simulink model "DynamicModelRacingWind"  (R2016b)
settings: configuration reference "WheelSimConfiguration2016" (kept outside this file)
settings Model: Creator=At  LastModifiedBy=At
settings ConfigSetRef: SourceLocation=Base Workspace

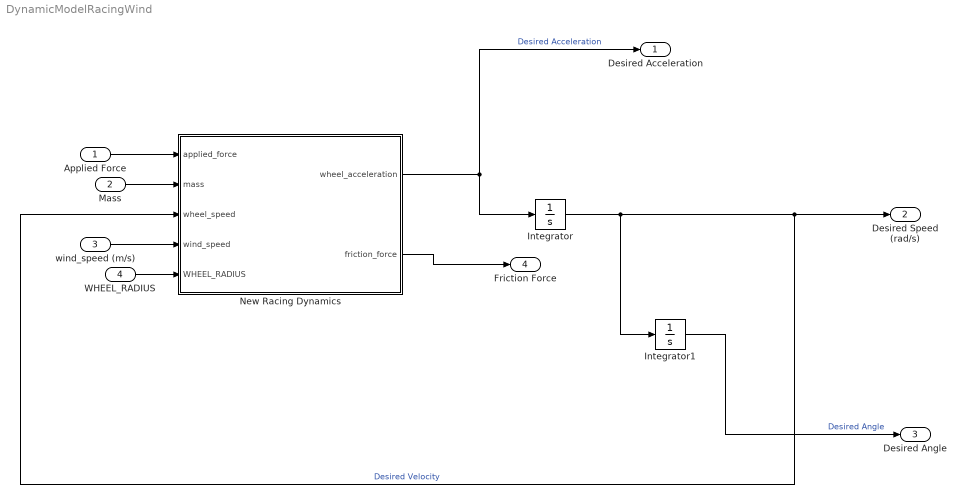
== system DynamicModelRacingWind ==
  Applied Force : Inport
  Mass : Inport  Port=2
  wind_speed (m/s) : Inport  Port=3
  WHEEL_RADIUS : Inport  Port=4
  Integrator : Integrator
  Integrator1 : Integrator
  New Racing Dynamics : MATLAB Function  TreatAsAtomicUnit=on
  Desired Acceleration : Outport
  Desired Speed (rad/s) : Outport  Port=2
  Desired Angle : Outport  Port=3
  Friction Force : Outport  Port=4
  wires:
  New Racing Dynamics/1(wheel_acceleration) -> Integrator/1, Desired Acceleration/1  "Desired Acceleration"
  Integrator/1 -> Desired Speed (rad/s)/1, New Racing Dynamics/3(wheel_speed), Integrator1/1  "Desired Velocity"
  Integrator1/1 -> Desired Angle/1  "Desired Angle"
  WHEEL_RADIUS/1 -> New Racing Dynamics/5(WHEEL_RADIUS)
  wind_speed (m/s)/1 -> New Racing Dynamics/4(wind_speed)
  Mass/1 -> New Racing Dynamics/2(mass)
  Applied Force/1 -> New Racing Dynamics/1(applied_force)
  New Racing Dynamics/2(friction_force) -> Friction Force/1

== matlab function DynamicModelRacingWind/New Racing Dynamics ==
  data: applied_force input; wheel_acceleration output; mass input; wheel_speed input; wind_speed input; WHEEL_RADIUS input; friction_force output
function [wheel_acceleration, friction_force]  = dynamics(applied_force, mass, wheel_speed, wind_speed,  WHEEL_RADIUS)

%% This function calculates the wheel acceleration based on the new dynamic model of propelling in a straight line. 


wheel_speed_m=wheel_speed*WHEEL_RADIUS; % converts wheel speed to m/s

friction_force= (0.05881229*mass+ 0.00766823*mass*wheel_speed_m+ 1.01871476*(wheel_speed_m-wind_speed)^2); %N

wheelchair_linear_acceleration = (applied_force - (friction_force * sign(wheel_speed))) / mass;

wheel_acceleration = wheelchair_linear_acceleration / WHEEL_RADIUS;
